simulink model "lineChanging"  (R2017a)
settings: Solver=VariableStepAuto  StartTime=0  StopTime=60  MaxStep=0.05  RelTol=1e-3
model workspace (MAT data in the model file):
  MCOS : class17 (value not decoded)
  LANE_NUM = 4
  LANE_WIDTH = 1
  MCOS : class17 (value not decoded)
  ROAD_WIDTH = 4
  MCOS : class17 (value not decoded)
  WORLD_SIZE = 12
  MCOS : class17 (value not decoded)
values from neighbouring files (symbols this model uses):
  m = rt.find('-isa','Simulink.BlockDiagram','-and','Name',mdl)    [configModel.m]
undefined symbols (not defined in the file or in its folder): n
(part 2 of 2)

== stateflow chart lineChanging/vehicle6 ==
  state Straight
    en:
    safeDist = max(norm(V(:,this))*1,MIN_SAFE_DIST);
    du:
    safeDist = max(norm(V(:,this))*1,MIN_SAFE_DIST);
    state Follow
      en:
      [dxfr, dvfr] = frontCarInfo();
      du:
      [dxfr, dvfr] = frontCarInfo();
      state Safe
        du:
        if dvfr < 0
        accelerateDrive();
        else
        slowDownDrive();
        end
      state Dangerous
        du:
        slowDownDrive();
      Safe -> Dangerous : [dxfr < 1.6*safeDist]
      Dangerous -> Safe : [dxfr > 2*safeDist]
      (default) -> Dangerous [order 2]
      (default) -> Safe [order 1] : [dxfr > 2*safeDist]
    state FreeDriving
      state Accelerate
        du:
        accelerateDrive();
      state FixRate
        en:
        setRateTo(V_MAX);
        du:
        fixedRateDrive();
      (default) -> Accelerate [order 2]
      Accelerate -> FixRate : [reach(V_MAX)]
      (default) -> FixRate [order 1] : [reach(V_MAX)]
    (default) -> Follow [order 1] : [hasFrontCar()]
    (default) -> FreeDriving [order 2]
    FreeDriving -> Follow : [hasFrontCar()]
    Follow -> FreeDriving : [frontCarHasLeft()]
  data: res function_output; res function_output; res function_output; target function_input; target function_input; dx function_output; dv function_output; idx function_output; X data_store_memory; this local uint8 size=1 =uint8(6); A_MAX constant double =2.5; D data_store_memory; V_MAX constant double =3; V data_store_memory; MIN_SAFE_DIST parameter; WORLD_SIZE parameter; dt parameter; dxfr local; dvfr local; safeDist local; FARAWAY parameter
  function slowDownDrive:
    | function slowDownDrive
    |  
    | x = X(:,this);
    | v = V(:,this);
    | a = D(:,this) * (-A_MAX);
    | 
    | x = x + v * dt + 0.5 * a * dt * dt;
    | v = v + a * dt;
    | 
    | % a rounded world
    | if x(1) > WORLD_SIZE
    |     x(1) = -WORLD_SIZE;
    | elseif x(1) < -WORLD_SIZE
    |     x(1) = WORLD_SIZE;
    | elseif x(2) > WORLD_SIZE
    |     x(2) = -WORLD_SIZE;
    | elseif x(2) < -WORLD_SIZE
    |     x(2) = WORLD_SIZE;
    | end
    | 
    | X(:,this) = x;
    | V(:,this) = v;
  function res = hasFrontCar:
    | function res = hasFrontCar
    | 
    | % constants
    | THRES = 2.25 * safeDist;
    | RANGE = 2 * WORLD_SIZE;
    | 
    | res = false;
    | 
    | % row of X: coordinate, col of X: num of cars
    | num = size(X, 2);
    | if num == 1
    |     return;
    | end
    | 
    | dx = ones(num, 1)*FARAWAY;
    | x = X(:,this);
    | d = D(:,this);
    | carSize = [0.3; 0.4];
    | 
    | for k=1:length(dx)
    |     
    |     if k ~= this
    |         % compute difference
    |         xdelta = X(:,k) - x;
    |     
    |         % parallel and vertical distance
    |         delta_p = dot(xdelta, d);
    |         delta_v = norm(xdelta - (d * delta_p));
    |     
    |         % vertical distance is larger than car width
    |         if delta_v < carSize(1)
    |             dx(k) = delta_p;
    |       
    |             % a rounded world
    |             dx(k) = mod((dx(k)+RANGE), RANGE);
    |         end
    |     end
    | end
    | 
    | % set zero dX to a large enough value
    | closest = min(dx);
    | res = closest <= THRES;
  function res = frontCarHasLeft:
    | function res = frontCarHasLeft
    | 
    | % Constants 
    | THRES = 2.5 * safeDist;
    | RANGE = 2 * WORLD_SIZE;
    | 
    | % if only one car in the environment return directly
    | res = true;
    | num = size(X, 1);
    | if num == 1
    |     return;
    | end
    | 
    | % get the closet car index and its distance
    | dx = zeros(num, 1);
    | x = X(:,this);
    | d = D(:,this);
    | car_size = [0.3; 0.4];
    | 
    | for k=1:length(dx)
    |     
    |     xdelta = X(:,k) - x;
    |     xdelta_p = dot(xdelta, d);                  % parallel component
    |     xdelta_v = norm(xdelta - (d * xdelta_p));   % vertical component
    |     
    |     % when the vertical component is larger than the car width
    |     if xdelta_v < car_size(1)
    |         dx(k) = xdelta_p;
    |         % since we are in the round world, normalize the distance if the 
    |         % front car is behind us 
    |         % a rounded world
    |         dx(k) = mod((dx(k)+RANGE), RANGE);
    |     else
    |         dx(k) = FARAWAY;
    |     end
    | end
    | 
    | % set the zero dx to a large enough value for convenience
    | dx(dx == 0) = FARAWAY;
    | closest = min(dx);
    | res = closest > THRES;
  function res = reach(target):
    | function res = reach(target)
    | 
    | res = abs(target - norm(V(:,this))) < 0.125;
  function accelerateDrive:
    | function accelerateDrive
    | 
    | x = X(:,this);
    | v = V(:,this);
    | a = D(:,this) * A_MAX;
    | 
    | x = x + v * dt + 0.5 * a * dt * dt;
    | v = v + a * dt;
    | 
    | % a rounded world
    | if x(1) > WORLD_SIZE
    |     x(1) = -WORLD_SIZE;
    | elseif x(1) < -WORLD_SIZE
    |     x(1) = WORLD_SIZE;
    | elseif x(2) > WORLD_SIZE
    |     x(2) = -WORLD_SIZE;
    | elseif x(2) < -WORLD_SIZE
    |     x(2) = WORLD_SIZE;
    | end
    | 
    | X(:,this) = x;
    | V(:,this) = v;
  function fixedRateDrive:
    | function fixedRateDrive
    | 
    | x = X(:,this);
    | v = V(:,this);
    | 
    | % update new position
    | x = x + v * dt;
    | 
    | % a rounded world
    | if x(1) > WORLD_SIZE
    |     x(1) = -WORLD_SIZE;
    | elseif x(1) < -WORLD_SIZE
    |     x(1) = WORLD_SIZE;
    | elseif x(2) > WORLD_SIZE
    |     x(2) = -WORLD_SIZE;
    | elseif x(2) < -WORLD_SIZE
    |     x(2) = WORLD_SIZE;
    | end
    | 
    | X(:,this) = x;
  function setRateTo(target):
    | function setRateTo(target)
    | 
    | V(:,this) = D(:,this) * target;
  function [dx,dv] = frontCarInfo:
    | function [dx,dv] = frontCarInfo()
    | 
    | index = frontCarIndex();
    | 
    | x = X(:,this);
    | v = V(:,this);
    | d = D(:,this);
    | 
    | xfront = X(:,index);
    | vfront = V(:,index);
    | 
    | range = 2 * WORLD_SIZE;
    | 
    | dx = mod((dot(xfront - x, d)+range), range);
    | dv = dot(vfront-v, d);
    | 
    | end
  function idx = frontCarIndex:
    | function idx = frontCarIndex
    | 
    | RANGE = 2*WORLD_SIZE;
    | 
    | dx = ones(size(X, 2), 1)*FARAWAY;
    | x = X(:,this);
    | v = V(:,this);
    | d = D(:,this);
    | 
    | for k=1:length(dx)
    |     xk = X(:,k);
    |     if k ~= this && (abs(xk(2)-x(2)) < 1)
    |         dx(k) = dot(xk - x, d);
    |         dx(k) = mod((dx(k)+RANGE), RANGE);
    |     end
    | end
    | 
    | % set zero dx to a large enough value
    | [~, idx] = min(dx);
    | idx = uint8(idx);
    | 
    | end

== stateflow chart lineChanging/Agent ==
  state HighLevelLogic [parallel]
    settings: executionOrder=2
    state Wait
    state CoolDown
    (default) -> HighLevelLogic.Wait
    HighLevelLogic.Wait -> CoolDown : [in(Moving.Straight.HasFrontCar)]
        | {CUTOFF.data = nextMove()
        | send(CUTOFF);}
    CoolDown -> HighLevelLogic.Wait : after(2, sec)
  state Moving [parallel]
    en:
    safeDistFront = max(norm(V(:,this))*SAFE_FACTOR,MIN_SAFE_DIST);
    du:
    safeDistFront = max(norm(V(:,this))*SAFE_FACTOR,MIN_SAFE_DIST);
    settings: executionOrder=1
    state Straight
      state HasFrontCar
        en:
        [dxfr, dvfr] = frontCarInfo();
        du:
        [dxfr, dvfr] = frontCarInfo();
        state Follow
          state AccSlightly
            en:
            GAS.data(1) = ...
            norm(V(:,this)) - dvfr;
            send(GAS);
          state SameRate
          state SlowDownSlightly
            en:
            BRAKE.data(1) = ...
            norm(V(:,this)) - dvfr;
            send(BRAKE);
          state Wait
          (default) -> (junction 196)
          (junction 196) -> Moving.Straight.HasFrontCar.Follow.SameRate [order 3]
          (junction 196) -> Moving.Straight.HasFrontCar.Follow.AccSlightly [order 1] : [dvfr < 0]
          Moving.Straight.HasFrontCar.Follow.Wait -> (junction 196) : after(0.5, sec)
          (junction 196) -> Moving.Straight.HasFrontCar.Follow.SlowDownSlightly [order 2] : [dvfr > 0]
          Moving.Straight.HasFrontCar.Follow.AccSlightly -> Moving.Straight.HasFrontCar.Follow.Wait
          Moving.Straight.HasFrontCar.Follow.SlowDownSlightly -> Moving.Straight.HasFrontCar.Follow.Wait
        state Dangerous
          en:
          BRAKE.data(1) = V_MIN;
          send(BRAKE);
        Moving.Straight.HasFrontCar.Dangerous -> Moving.Straight.HasFrontCar.Follow : [dxfr > 1*safeDistFront]
        Moving.Straight.HasFrontCar.Follow -> Moving.Straight.HasFrontCar.Dangerous : [dxfr < 0.5*safeDistFront]
        (default) -> Moving.Straight.HasFrontCar.Follow [order 1] : [dxfr > 1*safeDistFront]
        (default) -> Moving.Straight.HasFrontCar.Dangerous [order 2]
      state FreeDriving
        state Accelerate
          en:
          GAS.data(1) = V_MAX;
          send(GAS);
        state FixRate
        (default) -> Accelerate [order 2]
        Accelerate -> FixRate : [higherThan(V_MAX)]
        (default) -> FixRate [order 1] : [higherThan(V_MAX)]
      (default) -> Moving.Straight.HasFrontCar [order 1] : [hasFrontCar]
      (default) -> FreeDriving [order 2]
      FreeDriving -> Moving.Straight.HasFrontCar : [hasFrontCar]
      Moving.Straight.HasFrontCar -> FreeDriving : [frontCarHasLeft]
    state Init
      en:
      GAS.data = [0;0];
      BRAKE.data = [0;0];
      SHIFT.data = [0;0];
    state SlowDownToChange
    state LaneChange
      state Shift
        en:
        SHIFT.data = [yend; ystart];
        send(SHIFT);
      state WaitDuringShift
      (default) -> Shift
      WaitDuringShift -> Shift : [alwaysFalse()]
      Shift -> WaitDuringShift : [alwaysFalse()]
    state WaitForLaneChange
      state HasFrontCar
        en:
        [dxfr, dvfr] = frontCarInfo();
        du:
        [dxfr, dvfr] = frontCarInfo();
        state Follow
          state AccSlightly
            en:
            GAS.data(1) = ...
            norm(V(:,this)) - dvfr;
            send(GAS);
          state SameRate
          state SlowDownSlightly
            en:
            BRAKE.data(1) = ...
            norm(V(:,this)) - dvfr;
            send(BRAKE);
          state Wait
          (default) -> (junction 296)
          (junction 296) -> Moving.WaitForLaneChange.HasFrontCar.Follow.SameRate [order 3]
          (junction 296) -> Moving.WaitForLaneChange.HasFrontCar.Follow.AccSlightly [order 1] : [dvfr < 0]
          Moving.WaitForLaneChange.HasFrontCar.Follow.Wait -> (junction 296) : after(0.5, sec)
          (junction 296) -> Moving.WaitForLaneChange.HasFrontCar.Follow.SlowDownSlightly [order 2] : [dvfr > 0]
          Moving.WaitForLaneChange.HasFrontCar.Follow.AccSlightly -> Moving.WaitForLaneChange.HasFrontCar.Follow.Wait
          Moving.WaitForLaneChange.HasFrontCar.Follow.SlowDownSlightly -> Moving.WaitForLaneChange.HasFrontCar.Follow.Wait
        state Dangerous
          en:
          BRAKE.data(1) = V_MIN;
          send(BRAKE);
        Moving.WaitForLaneChange.HasFrontCar.Dangerous -> Moving.WaitForLaneChange.HasFrontCar.Follow : [dxfr > 1*safeDistFront]
        Moving.WaitForLaneChange.HasFrontCar.Follow -> Moving.WaitForLaneChange.HasFrontCar.Dangerous : [dxfr < 0.5*safeDistFront]
        (default) -> Moving.WaitForLaneChange.HasFrontCar.Follow [order 1] : [dxfr > 1*safeDistFront]
        (default) -> Moving.WaitForLaneChange.HasFrontCar.Dangerous [order 2]
      state FixedRate
      (default) -> Moving.WaitForLaneChange.HasFrontCar [order 1] : [hasFrontCar]
      (default) -> FixedRate [order 2]
      FixedRate -> Moving.WaitForLaneChange.HasFrontCar : [hasFrontCar]
      Moving.WaitForLaneChange.HasFrontCar -> FixedRate : [frontCarHasLeft]
    Moving.WaitForLaneChange -> Straight [order 1] : after(TIMEOUT, sec)
    Init -> Straight
    (junction 130) -> Straight
    Straight -> (junction 128) : CUTOFF
        | {decision = CUTOFF.data;}
    LaneChange -> Straight : [completeLaneChange()]
    (default) -> Init
    (junction 128) -> (junction 130) [order 1] : [decision == Decision.Straight]
    (junction 128) -> (junction 229) [order 2]
    (junction 229) -> SlowDownToChange [order 2]
    (junction 229) -> Moving.WaitForLaneChange [order 1] : [higherThan(V_CHANGE)]
        | {prepLaneChange(decision);}
    Moving.WaitForLaneChange -> LaneChange [order 3] : [decision == Decision.Left && ...
        | leftLaneClear()]
    Moving.WaitForLaneChange -> LaneChange [order 2] : [decision == Decision.Right && ...
        | rightLaneClear()]
  state WaitForLaneChange [parallel] [commented out]
    en:
    [hasfr, vfr] = leftFrontCarRate();
    v = norm(V(:,this));
    du:
    v = norm(V(:,this));
    state Acc [commented out]
      en:
      GAS.data(1) = ...
      V_MAX;
      send(GAS);
    state SlowDown [commented out]
      en:
      BRAKE.data(1) = ...
      V_CHANGE;
      send(BRAKE);
    state fixedRate [commented out]
    (default) -> (junction 177) [commented out]
    (junction 177) -> (junction 182) [commented out]
    (junction 182) -> Acc [commented out] : [vfr < V_MAX]
    (junction 182) -> (junction 180) [commented out]
    (junction 177) -> (junction 180) [commented out] : [hasFrontCar]
    Acc -> (junction 180) [commented out] : [hasFrontCar]
    (junction 180) -> SlowDown [commented out]
    Acc -> fixedRate [commented out] : [higherThan(vfr)]
    SlowDown -> fixedRate [commented out] : [lowerThan(V_CHANGE)]
    (default) -> fixedRate [commented out] : [~hasfr]
  data: dxfr local; dvfr local; dxfr local; dvfr local; target function_input; res function_output; res function_output; res function_output; res function_output; target function_input; dx function_output; dv function_output; idx function_output; res function_output; goal function_input; vfr local double size=1; hasfr local; v local; res function_output; res function_output; res function_output; res function_output; velocity function_output; res function_output; X data_store_memory; this local uint8 size=1 =uint8(1); D data_store_memory; V_MAX constant double =4; V data_store_memory; MIN_SAFE_DIST parameter; WORLD_SIZE parameter; dt parameter; safeDistFront local; FARAWAY parameter; yend local; ystart local; LANE_NUM parameter; ROAD_WIDTH parameter; decision local Enum: Decision =Decision.Left; BRAKE output; GAS output; SHIFT output; V_CHANGE constant double =1.25; V_MIN constant double =0.125; CUTOFF local Enum: Decision size=1; TIMEOUT constant double =5; SAFE_FACTOR parameter
  function res = lowerThan(target):
    | function res = lowerThan(target)
    |  
    | v_norm = norm(V(:,this));
    | 
    | res = (v_norm <= target) || ((norm(V(:,this))-target) < 0.125);
  function res = hasFrontCar:
    | function res = hasFrontCar
    | 
    | % constants
    | THRES = 1.5 * safeDistFront;
    | RANGE = 2 * WORLD_SIZE;
    | 
    | res = false;
    | 
    | % row of X: coordinate, col of X: num of cars
    | num = size(X, 2);
    | if num == 1
    |     return;
    | end
    | 
    | dx = ones(num, 1)*FARAWAY;
    | x = X(:,this);
    | d = D(:,this);
    | carSize = [0.3; 0.4];
    | 
    | for k=1:length(dx)
    |     
    |     if k ~= this
    |         % compute difference
    |         xdelta = X(:,k) - x;
    |     
    |         % parallel and vertical distance
    |         delta_p = dot(xdelta, d);
    |         delta_v = norm(xdelta - (d * delta_p));
    |     
    |         % vertical distance is larger than car width
    |         if delta_v < carSize(1)
    |             dx(k) = delta_p;
    |       
    |             % a rounded world
    |             dx(k) = mod((dx(k)+RANGE), RANGE);
    |         end
    |     end
    | end
    | 
    | % set zero dX to a large enough value
    | closest = min(dx);
    | res = closest <= THRES;
  function res = frontCarHasLeft:
    | function res = frontCarHasLeft
    | 
    | % Constants 
    | THRES = 2 * safeDistFront;
    | RANGE = 2 * WORLD_SIZE;
    | 
    | % if only one car in the environment return directly
    | res = true;
    | num = size(X, 1);
    | if num == 1
    |     return;
    | end
    | 
    | % get the closet car index and its distance
    | dx = zeros(num, 1);
    | x = X(:,this);
    | d = D(:,this);
    | car_size = [0.3; 0.4];
    | 
    | for k=1:length(dx)
    |     
    |     xdelta = X(:,k) - x;
    |     xdelta_p = dot(xdelta, d);                  % parallel component
    |     xdelta_v = norm(xdelta - (d * xdelta_p));   % vertical component
    |     
    |     % when the vertical component is larger than the car width
    |     if xdelta_v < car_size(1)
    |         dx(k) = xdelta_p;
    |         % since we are in the round world, normalize the distance if the 
    |         % front car is behind us 
    |         % a rounded world
    |         dx(k) = mod((dx(k)+RANGE), RANGE);
    |     else
    |         dx(k) = FARAWAY;
    |     end
    | end
    | 
    | % set the zero dx to a large enough value for convenience
    | dx(dx == 0) = FARAWAY;
    | closest = min(dx);
    | res = closest > THRES;
  function res = higherThan(target):
    | function res = higherThan(target)
    | 
    | v_norm = norm(V(:,this));
    | 
    | res = (v_norm >= target) || ((target - norm(V(:,this))) < 0.125);
  function [dx,dv] = frontCarInfo:
    | function [dx,dv] = frontCarInfo()
    | 
    | index = frontCarIndex();
    | 
    | x = X(:,this);
    | v = V(:,this);
    | d = D(:,this);
    | 
    | xfront = X(:,index);
    | vfront = V(:,index);
    | 
    | range = 2 * WORLD_SIZE;
    | 
    | dx = mod((dot(xfront - x, d)+range), range);
    | dv = dot(vfront-v, d);
    | 
    | end
  function idx = frontCarIndex:
    | function idx = frontCarIndex
    | 
    | RANGE = 2*WORLD_SIZE;
    | 
    | dx = ones(size(X, 2), 1)*FARAWAY;
    | x = X(:,this);
    | v = V(:,this);
    | d = D(:,this);
    | 
    | for k=1:length(dx)
    |     xk = X(:,k);
    |     if k ~= this && (abs(xk(2)-x(2)) < 1)
    |         dx(k) = dot(xk - x, d);
    |         dx(k) = mod((dx(k)+RANGE), RANGE);
    |     end
    | end
    | 
    | % set zero dx to a large enough value
    | [~, idx] = min(dx);
    | idx = uint8(idx);
    | 
    | end
  function res = rightLaneClear:
    | function res = rightLaneClear
    | 
    | res = true;
    | 
    | lnum = LANE_NUM;
    | rwidth = ROAD_WIDTH;
    | range = 2*WORLD_SIZE;
    | 
    | x = X(:,this);
    | v = V(:,this);
    | 
    | pos_y = FARAWAY*ones(20, 1);
    | if mod(lnum,2) == 0
    |     k = (-1*(rwidth/2-0.5));
    |     for i=1:lnum
    |         pos_y(i) = k;
    |         k = k + 1;
    |     end
    | else
    |     k = (-1*(rwidth/2));
    |     for i=1:lnum
    |         pos_y(i) = k;
    |         k = k + 1;
    |     end
    | end
    | 
    | [~, index] = min(abs(pos_y-x(2)));
    | if index == 1
    |     res = false;
    |     
    |     % TODO: change the planning to demo different scenario
    |     
    |     return;
    | end
    | 
    | ys = X(2,:)-x(2);
    | ys(this) = FARAWAY;
    | indices = find(ys < 0 & ys >= -1);  
    | if isempty(indices)
    |     return;
    | end
    | 
    | for i = 1:length(indices)
    |     
    |     idx = indices(i);
    |     xb = X(:,idx);
    |     vb = V(:,idx);
    |     
    |     dx = mod(x(1)+range-xb(1), range);
    |     dv = v(1) - vb(1);
    |     
    |     backSafeDist = max(SAFE_FACTOR*vb(1), MIN_SAFE_DIST);
    | 
    |     % front car 
    |     if dx >= range - 0.5*safeDistFront
    |         res = false;
    |     % the car in the behind is too close
    |     elseif dx <= backSafeDist
    |         res = false;
    |     % the distance is larger than safeDist but current speed is too slow
    |     elseif dx <= 1.5*backSafeDist && dv < 0
    |         disp(1.5*backSafeDist);
    |         res = false;
    |     end
    | end
  function prepLaneChange(goal):
    | function prepLaneChange(goal)
    |  
    | x = X(:,this);
    | ystart = x(2);
    | 
    | if goal == Decision.Left
    |     yend = x(2)+1;
    | elseif goal == Decision.Right
    |     yend = x(2)-1;
    | else
    |     error('Go straight decision is not allowed here');
    | end
  function res = completeLaneChange:
    | function res = completeLaneChange
    |  
    | x = X(:,this);
    | 
    | res = abs(yend - x(2)) == 0;
  function res = leftLaneClear:
    | function res = leftLaneClear
    |  
    | res = true;
    | 
    | lnum = LANE_NUM;
    | rwidth = ROAD_WIDTH;
    | range = 2*WORLD_SIZE;
    | 
    | x = X(:,this);
    | v = V(:,this);
    | 
    | pos_y = FARAWAY*ones(20, 1);
    | if mod(lnum,2) == 0
    |     k = (-1*(rwidth/2-0.5));
    |     for i=1:lnum
    |         pos_y(i) = k;
    |         k = k + 1;
    |     end
    | else
    |     k = (-1*(rwidth/2));
    |     for i=1:lnum
    |         pos_y(i) = k;
    |         k = k + 1;
    |     end
    | end
    | 
    | [~, index] = min(abs(pos_y-x(2)));
    | if index == lnum
    |     res = false;
    |     
    |     % TODO: change the planning to demo different scenario
    |     
    |     return;
    | end
    | 
    | ys = X(2,:)-x(2);
    | ys(this) = FARAWAY;
    | indices = find(ys > 0 & ys <= 1);  
    | if isempty(indices)
    |     return;
    | end
    | 
    | for i = 1:length(indices)
    |     
    |     idx = indices(i);
    |     xb = X(:,idx);
    |     vb = V(:,idx);
    |     
    |     dx = mod(x(1)+range-xb(1), range);
    |     dv = v(1) - vb(1);
    |     
    |     safeDistBack = max(SAFE_FACTOR*vb(1), MIN_SAFE_DIST);
    | 
    |     % front car 
    |     if dx >= range - safeDistFront
    |         res = false;
    |     % the car in the behind is too close
    |     elseif dx <= safeDistBack
    |         res = false;
    |     % the distance is larger than safeDist but current speed is too slow
    |     elseif dx <= 1.5*safeDistBack && dv < 0
    | %         disp(1.5*safeDistBack);
    |         res = false;
    |     end
    | end
  function res = alwaysFalse:
    | function res = alwaysFalse
    | 
    | res = false;
  function [res, velocity] = leftFrontCarRate:
    | function [res, velocity] = leftFrontCarRate
    | 
    | res = false;
    | velocity = -1;
    |  
    | % fetch environment variables
    | lnum = LANE_NUM;
    | rwidth = ROAD_WIDTH;
    | range = 2*WORLD_SIZE;
    | 
    | x = X(:,this);
    | v = V(:,this);
    | 
    | pos_y = FARAWAY*ones(20, 1);
    | if mod(lnum,2) == 0
    |     k = (-1*(rwidth/2-0.5));
    |     for i=1:lnum
    |         pos_y(i) = k;
    |         k = k + 1;
    |     end
    | else
    |     k = (-1*(rwidth/2));
    |     for i=1:lnum
    |         pos_y(i) = k;
    |         k = k + 1;
    |     end
    | end
    | 
    | [~, index] = min(abs(pos_y-x(2)));
    | if index == lnum
    |     return;
    | end
    | 
    | ys = X(2,:)-x(2);
    | ys(this) = FARAWAY;
    | indices = find(ys > 0 & ys <= 1);  
    | if isempty(indices)
    |     disp('no car on the adjacent lane');
    | end
    | 
    | for i = 1:length(indices)
    |     
    |     idx = indices(i);
    |     xb = X(:,idx);
    |     vb = V(:,idx);
    |     dx = mod(x(1)+range-xb(1), range);
    | 
    |     % front car 
    |     if dx >= range - 0.5*safeDistFront
    |         res = true;
    |         velocity = norm(vb);
    |     end
    | end
  function res = nextMove:
    | function res = nextMove
    | 
    | res = Decision.Straight;
    | 
    | x = X(:,this);
    | v = V(:,this);
    | 
    | % compute environment par
    | lnum = LANE_NUM;
    | rwidth = ROAD_WIDTH;
    | range = 2*WORLD_SIZE;
    | pos_y = FARAWAY*ones(20, 1);
    | if mod(lnum,2) == 0
    |     k = (-1*(rwidth/2-0.5));
    |     for i=1:lnum
    |         pos_y(i) = k;
    |         k = k + 1;
    |     end
    | else
    |     k = (-1*(rwidth/2));
    |     for i=1:lnum
    |         pos_y(i) = k;
    |         k = k + 1;
    |     end
    | end
    | 
    | checkLeft = true;
    | checkRight = true;
    | 
    | % identify the current lane 
    | [~, index] = min(abs(pos_y-x(2)));
    | if index == lnum
    |     % on the left-most lane
    |     disp('no check on left');
    |     checkLeft = false;
    | elseif index == 1
    |     % on the right-most lane
    |     disp('no check on right');
    |     checkRight = false;
    | end
    | 
    | % check whether the lane is occupied
    | ys = X(2,:)-x(2);
    | ys(this) = FARAWAY;
    | leftLaneCars = find(ys > 0 & ys <= 1);
    | rightLaneCars = find(ys < 0 & ys >= -1);
    | if checkLeft && isempty(leftLaneCars)
    |     res = Decision.Left;
    |     return;
    | elseif checkRight && isempty(rightLaneCars)
    |     res = Decision.Right;
    |     return;
    | end
    | 
    | % check whether the safe distance is large enough
    | if checkLeft
    |     isClear = true;
    |     disp('checking left');
    |     for i = 1:length(leftLaneCars)
    |         
    |         idx = leftLaneCars(i);
    |         xb = X(:,idx);
    |         vb = V(:,idx);
    |     
    |         dx = mod(x(1)+range-xb(1), range);
    |         dv = v(1) - vb(1);
    |     
    |         safeDistBack = max(SAFE_FACTOR*vb(1), MIN_SAFE_DIST);
    | 
    |         if dx >= range - safeDistFront
    |             % front car
    |             disp('left front');
    |             isClear = false;
    |         elseif dx <= safeDistBack
    |             % the car in the behind is too close
    |             disp('left close');
    |             isClear = false;
    |         elseif dx <= 1.5*safeDistBack && dv < 0
    |             % the distance is larger than safeDist but current speed is too slow
    |             disp('left but you are slow');
    |             isClear = false;
    |         end
    |     end
    |     
    |     if isClear
    |         res = Decision.Left;
    |         return;
    |     end
    | end
    | 
    | % check whether the safe distance is large enough
    | if checkRight
    |     isClear = true;
    |     disp('checking right');
    |     for i = 1:length(rightLaneCars)
    |     
    |         idx = rightLaneCars(i);
    |         xb = X(:,idx);
    |         vb = V(:,idx);
    |     
    |         dx = mod(x(1)+range-xb(1), range);
    |         dv = v(1) - vb(1);
    |     
    |         safeDistBack = max(SAFE_FACTOR*vb(1), MIN_SAFE_DIST);
    |  
    |         if dx >= range - safeDistFront
    |             % front car
    |             disp('right front');
    |             isClear = false;
    |         elseif dx <= safeDistBack
    |             % the car in the behind is too close
    |             disp('right close');
    |             isClear = false;
    |         elseif dx <= 1.5*safeDistBack && dv < 0
    |             % the distance is larger than safeDist but current speed is too slow
    |             disp('right but you are slow');
    |             isClear = false;
    |         end
    |     end
    |     
    |     if isClear
    |         res = Decision.Right;
    |     end
    | end
